simulink model "planarBAT_th"  (R2018b)
settings: Solver=VariableStepAuto  StartTime=0.0  StopTime=10.0  RelTol=1e-3
libraries: planarBAT_ul x1
settings Model: Creator=Ayaz  LastModifiedBy=Ayaz

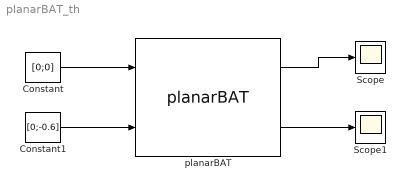
== system planarBAT_th ==
  Constant : Constant  Value=[0;0]  VectorParams1D=off
  Constant1 : Constant  Value=[0;-0.6]  VectorParams1D=off
  Scope : Scope
  Scope1 : Scope
  planarBAT : planarBAT_ul/planarBAT  rhoF=1  gravAcc=1  mT=1  BF=1.5  Sref=1  Cd=0.5  ini_rCM=[0; 100]  ini_vCM=[0;0]
  wires:
  Constant/1 -> planarBAT/1
  Constant1/1 -> planarBAT/2
  planarBAT/1 -> Scope/1
  planarBAT/2 -> Scope1/1
